simulink model "chap1_2sim"  (Simulink 7.7)
settings: Solver=ode45  StartTime=0.0  StopTime=10  RelTol=1e-3
settings Model: Creator=liujk  LastModifiedBy=ljk  ExtModeTrigMode=oneshot  ExtModeArmWhenConnect=off
settings DataIOCC: LimitDataPoints=off  SignalLoggingName=sigsOut
settings OptimizationCC: BooleanDataType=off  ExpressionDepthLimit=128
settings DebuggingCC: SaveWithParameterizedLinksMsg=none  SignalResolutionControl=TryResolveAllWithWarning  SolverPrmCheckMsg=none  MultiTaskDSMMsg=warning  MultiTaskCondExecSysMsg=none  StrictBusMsg=None
settings HardwareCC: TargetUnknown=on
settings RTWCC: IncludeERTFirstTime=on
settings CodeAppCC: CustomSymbolStrType=$N$R$M_T

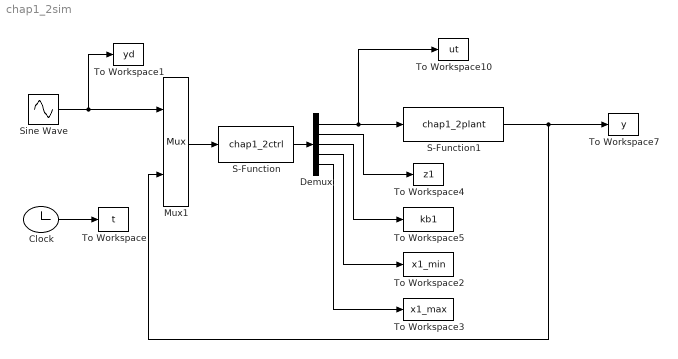
== system chap1_2sim ==
  Clock : Clock
  Demux : Demux  Outputs=5
  Mux1 : Mux  Inputs=2
  S-Function : S-Function  FunctionName=chap1_2ctrl  EnableBusSupport=off
  S-Function1 : S-Function  FunctionName=chap1_2plant  EnableBusSupport=off
  Sine Wave : Sin  SampleTime=0
  To Workspace : ToWorkspace  VariableName=t  SampleTime=-1  SaveFormat=Array
  To Workspace1 : ToWorkspace  VariableName=yd  SampleTime=-1  SaveFormat=Array
  To Workspace10 : ToWorkspace  VariableName=ut  SampleTime=-1  SaveFormat=Array
  To Workspace2 : ToWorkspace  VariableName=x1_min  SampleTime=-1  SaveFormat=Array
  To Workspace3 : ToWorkspace  VariableName=x1_max  SampleTime=-1  SaveFormat=Array
  To Workspace4 : ToWorkspace  VariableName=z1  SampleTime=-1  SaveFormat=Array
  To Workspace5 : ToWorkspace  VariableName=kb1  SampleTime=-1  SaveFormat=Array
  To Workspace7 : ToWorkspace  VariableName=y  SampleTime=-1  SaveFormat=Array
  wires:
  Mux1/1 -> S-Function/1
  S-Function1/1 -> Mux1/2, To Workspace7/1
  Sine Wave/1 -> Mux1/1, To Workspace1/1
  Clock/1 -> To Workspace/1
  S-Function/1 -> Demux/1
  Demux/1 -> S-Function1/1, To Workspace10/1
  Demux/2 -> To Workspace4/1
  Demux/3 -> To Workspace5/1
  Demux/4 -> To Workspace2/1
  Demux/5 -> To Workspace3/1
